simulink model "labc2_robusto_observador"  (R2023a)
settings: Solver=VariableStepAuto  StartTime=0.0  StopTime=5  RelTol=1e-3
values from neighbouring files (symbols this model uses):
  A = [-Ra/La -kg/La/kt; ka*kt/J -f/J]    [labc2_p2_final.m]    (also in robusto2_lc2.m = [[ -113.5203 -34.3792];[27.0249 -0.3312]]; robusto_labc2.m = [[ -113.5203 -34.3792];[27.0249 -0.3312]])
  b = [1/La;0]    [labc2_p2_final.m]    (also in robusto2_lc2.m = [46.6079 0]'; robusto_labc2.m = [46.6079 0]')
  c = [0 1]    [labc2_p2_final.m]    (also in robusto2_lc2.m; robusto_labc2.m)
  ki = k_total(3)    [labc2_p2_final.m]    (also in robusto2_lc2.m = k_robusto(end))
  kt_ee = place(A, b, polos)    [labc2_p2_final.m]    (also in robusto2_lc2.m = k_robusto(1:2); robusto_labc2.m)
settings Model: Creator=wesle  LastModifiedBy=wesle

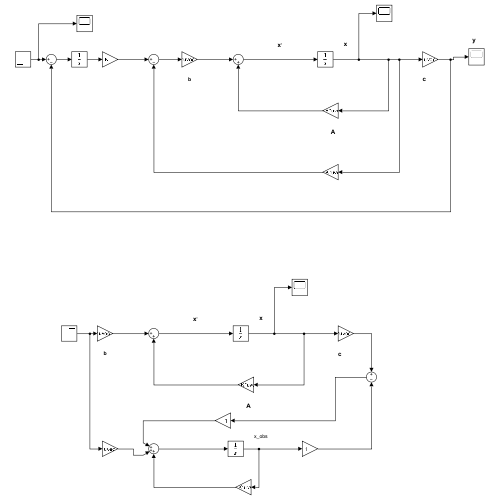
[thumbnail: Simulink's stored preview of the top-level diagram]
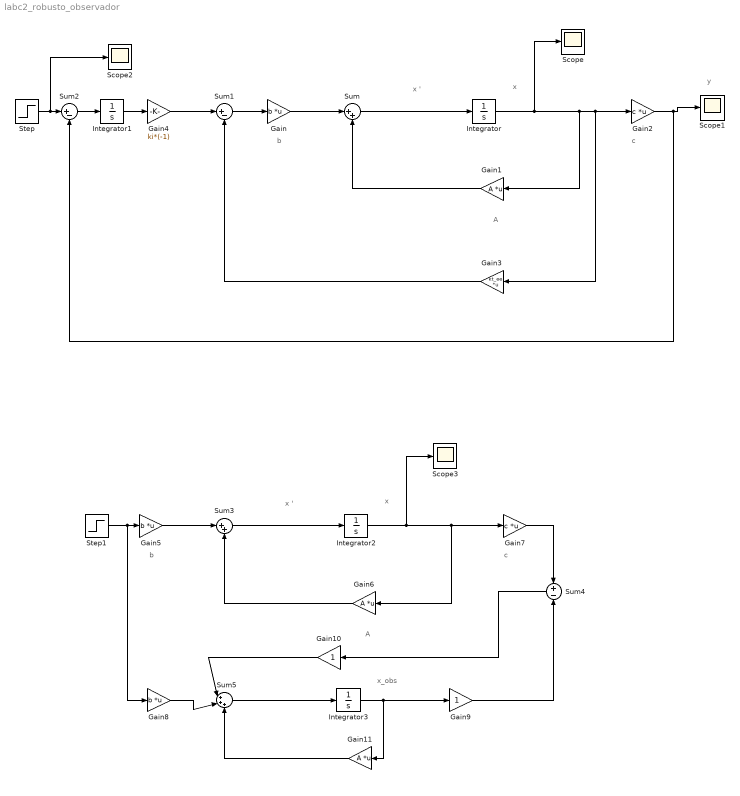
== system labc2_robusto_observador ==
  note: x_obs
  note: b
  note: c
  note: A
  note: x '
  note: x
  note: y
  note: b
  note: c
  note: A
  note: x '
  note: x
  Gain : Gain  Gain=b  Multiplication=Matrix(K*u) (u vector)
  Gain1 : Gain  Gain=A  Multiplication=Matrix(K*u) (u vector)
  Gain10 : Gain
  Gain11 : Gain  Gain=A  Multiplication=Matrix(K*u) (u vector)
  Gain2 : Gain  Gain=c  Multiplication=Matrix(K*u) (u vector)
  Gain3 : Gain  Gain=kt_ee  Multiplication=Matrix(K*u) (u vector)
  Gain4 : Gain  Gain=ki*(-1)
  Gain5 : Gain  Gain=b  Multiplication=Matrix(K*u) (u vector)
  Gain6 : Gain  Gain=A  Multiplication=Matrix(K*u) (u vector)
  Gain7 : Gain  Gain=c  Multiplication=Matrix(K*u) (u vector)
  Gain8 : Gain  Gain=b  Multiplication=Matrix(K*u) (u vector)
  Gain9 : Gain
  Integrator{,1..3} (4 alike) : Integrator
  Scope{,1..3} (4 alike) : Scope
  Step : Step  SampleTime=0
  Step1 : Step  SampleTime=0
  Sum : Sum  Inputs=|++
  Sum1 : Sum  Inputs=|+-
  Sum2 : Sum  Inputs=|+-
  Sum3 : Sum  Inputs=|++
  Sum4 : Sum  Inputs=+-
  Sum5 : Sum  Inputs=|+++
  wires:
  Sum/1 -> Integrator/1
  Gain/1 -> Sum/1
  Gain1/1 -> Sum/2
  Integrator/1 -> Scope/1, Gain1/1, Gain3/1, Gain2/1
  Gain2/1 -> Scope1/1, Sum2/2
  Gain3/1 -> Sum1/2
  Sum1/1 -> Gain/1
  Step/1 -> Scope2/1, Sum2/1
  Sum2/1 -> Integrator1/1
  Integrator1/1 -> Gain4/1
  Gain4/1 -> Sum1/1
  Sum3/1 -> Integrator2/1
  Gain5/1 -> Sum3/1
  Gain6/1 -> Sum3/2
  Step1/1 -> Gain8/1, Gain5/1
  Gain7/1 -> Sum4/1
  Integrator2/1 -> Scope3/1, Gain6/1, Gain7/1
  Integrator3/1 -> Gain11/1, Gain9/1
  Gain8/1 -> Sum5/2
  Gain10/1 -> Sum5/1
  Sum5/1 -> Integrator3/1
  Gain11/1 -> Sum5/3
  Gain9/1 -> Sum4/2
  Sum4/1 -> Gain10/1
